simulink model "Ej2_v2_1"  (R2015a)
settings: Solver=ode45  StartTime=0.0  StopTime=30  RelTol=1e-3
libraries: simulink x1, cstblocks x1
settings Model: Creator=Daniel  LastModifiedBy=Daniel

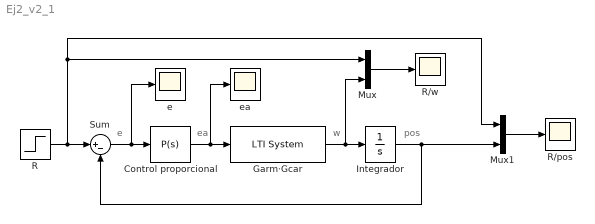
== system Ej2_v2_1 ==
  note: pos
  note: w
  note: e
  note: ea
  Control proporcional : simulink/Continuous/PID Controller  Controller=P  TimeDomain=Continuous-time  SampleTime=-1  IntegratorMethod=Forward Euler  FilterMethod=Forward Euler  Form=Ideal  UseFilter=on  ControllerParametersSource=internal  P=1  I=0  D=0  N=100  InitialConditionSource=internal  InitialConditionForIntegrator=0  InitialConditionForFilter=0  ExternalReset=none  LimitOutput=off  UpperSaturationLimit=12  LowerSaturationLimit=-inf  LinearizeAsGain=on  AntiWindupMode=none  Kb=1  TrackingMode=off  Kt=1  PParamMin=[]  PParamMax=[]  IParamMin=[]  IParamMax=[]  DParamMin=[]  DParamMax=[]  NParamMin=[]  NParamMax=[]  KbParamMin=[]  KbParamMax=[]  KtParamMin=[]  KtParamMax=[]  POutMin=[]  POutMax=[]  IOutMin=[]  IOutMax=[]  DOutMin=[]  DOutMax=[]  NOutMin=[]  NOutMax=[]  KbOutMin=[]  KbOutMax=[]  KtOutMin=[]  KtOutMax=[]  IntegratorOutMin=[]  IntegratorOutMax=[]  FilterOutMin=[]  FilterOutMax=[]  SumOutMin=[]  SumOutMax=[]  SumI1OutMin=[]  SumI1OutMax=[]  SumI2OutMin=[]  SumI2OutMax=[]  SumI3OutMin=[]  SumI3OutMax=[]  SumDOutMin=[]  SumDOutMax=[]  SaturationOutMin=[]  SaturationOutMax=[]  IntegratorContinuousStateAttributes=''  IntegratorStateMustResolveToSignalObject=off  IntegratorRTWStateStorageClass=Auto  FilterContinuousStateAttributes=''  FilterStateMustResolveToSignalObject=off  FilterRTWStateStorageClass=Auto  DifferentiatorICPrevScaledInput=0  DifferentiatorOutMin=[]  DifferentiatorOutMax=[]
  Garm·Gcar : cstblocks/LTI System  sys=G  IC=[]
  Integrador : Integrator
  Mux : Mux  Inputs=2
  Mux1 : Mux  Inputs=2
  R : Step  Time=0  After=0.6  SampleTime=0
  R/pos : Scope
      settings: SaveName=pos
  R/w : Scope
      settings: YMin=0  YMax=0.6  SaveName=w
  Sum : Sum  Inputs=|+-
  e : Scope
      settings: SaveName=e
  ea : Scope
      settings: SaveName=ea
  wires:
  Sum/1 -> e/1, Control proporcional/1
  Control proporcional/1 -> ea/1, Garm·Gcar/1
  Garm·Gcar/1 -> Mux/2, Integrador/1
  Integrador/1 -> Mux1/2, Sum/2
  Mux1/1 -> R/pos/1
  Mux/1 -> R/w/1
  R/1 -> Mux1/1, Mux/1, Sum/1
